simulink model "problem7"  (R2020a)
settings: Solver=VariableStepAuto  StartTime=0.0  StopTime=10.0  RelTol=1e-3
settings Model: Creator=HP  LastModifiedBy=HP

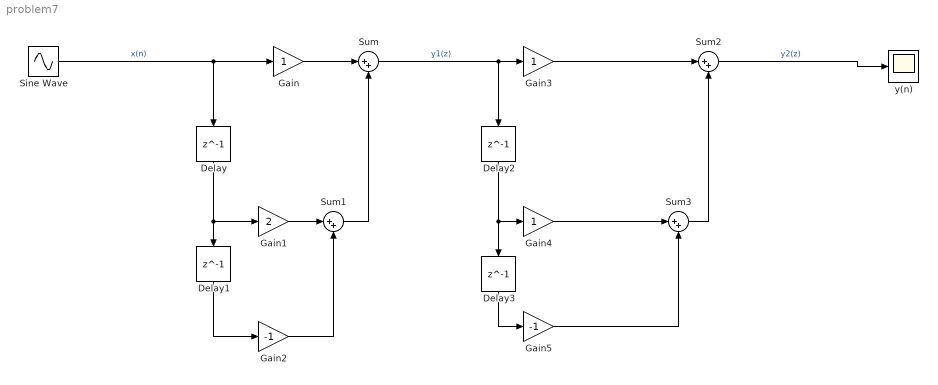
== system problem7 ==
  Delay{,1..3} (4 alike) : Delay  DelayLength=1  InitialCondition=0
  Gain : Gain
  Gain1 : Gain  Gain=2
  Gain2 : Gain  Gain=-1
  Gain3 : Gain
  Gain4 : Gain
  Gain5 : Gain  Gain=-1
  Sine Wave : Sin  SampleTime=0
  Sum{,1..3} (4 alike) : Sum  Inputs=|++
  y(n) : Scope
  wires:
  Sine Wave/1 -> Delay/1, Gain/1  "x(n)"
  Delay/1 -> Delay1/1, Gain1/1
  Sum1/1 -> Sum/2
  Sum/1 -> Gain3/1, Delay2/1  "y1(z)"
  Delay2/1 -> Gain4/1, Delay3/1
  Sum2/1 -> y(n)/1  "y2(z)"
  Sum3/1 -> Sum2/2
  Gain/1 -> Sum/1
  Gain1/1 -> Sum1/1
  Delay1/1 -> Gain2/1
  Gain2/1 -> Sum1/2
  Gain3/1 -> Sum2/1
  Gain4/1 -> Sum3/1
  Delay3/1 -> Gain5/1
  Gain5/1 -> Sum3/2
